simulink model "Signal_Generator"  (R2017a)
settings: Solver=VariableStepAuto  StartTime=0.0  StopTime=0.001  RelTol=1e-3
libraries: dspbuff3 x2
settings Model: Creator=Alam  LastModifiedBy=aparih

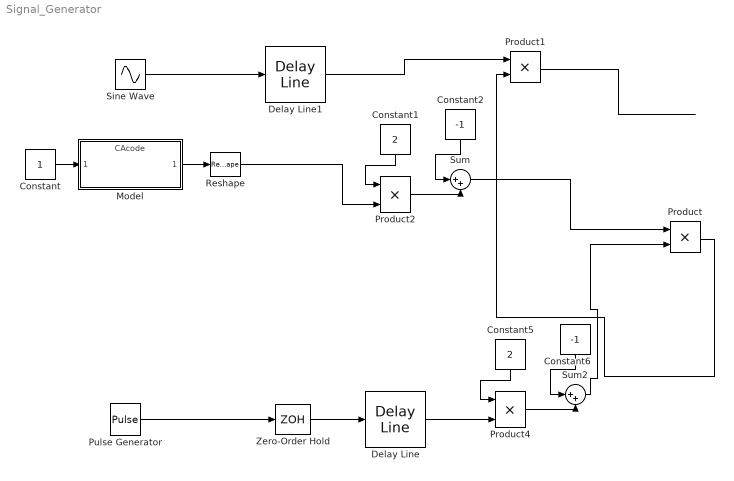
== system Signal_Generator ==
  Constant : Constant
  Constant1 : Constant  Value=2
  Constant2 : Constant  Value=-1
  Constant5 : Constant  Value=2
  Constant6 : Constant  Value=-1
  Delay Line : dspbuff3/Delay Line  siz=65536  ic=0  directfeed=off  enable_output=off  hold_output=off  OutputFrames=off
      settings: SourceProductName=DSP System Toolbox  SourceProductBaseCode=DS
  Delay Line1 : dspbuff3/Delay Line  siz=65536  ic=0  directfeed=off  enable_output=off  hold_output=off  OutputFrames=off
      settings: SourceProductName=DSP System Toolbox  SourceProductBaseCode=DS
  Model : ModelReference  ModelNameDialog=CAcode.mdl  SimulationMode=Normal  ModelReferenceVersion=1.40
  Product{,1..2,4} (4 alike) : Product
  Pulse Generator : DiscretePulseGenerator  PulseType=Time based  Period=0.0001  PulseWidth=50
  Reshape : Reshape  OutputDimensionality=Column vector (2-D)
  Sine Wave : Sin  Frequency=2*pi*9548000  Phase=pi/2  SampleTime=1.52587891e-8
  Sum : Sum  Inputs=|++
  Sum2 : Sum  Inputs=|++
  Zero-Order Hold : ZeroOrderHold  SampleTime=1.52587891e-8
  wires:
  Constant/1 -> Model/1
  Model/1 -> Reshape/1
  Constant1/1 -> Product2/1
  Product2/1 -> Sum/2
  Constant2/1 -> Sum/1
  Reshape/1 -> Product2/2
  Sine Wave/1 -> Delay Line1/1
  Sum2/1 -> Product/2
  Sum/1 -> Product/1
  Product/1 -> Product1/2
  Product1/1 -> ?
  Pulse Generator/1 -> Zero-Order Hold/1
  Constant6/1 -> Sum2/1
  Product4/1 -> Sum2/2
  Constant5/1 -> Product4/1
  Zero-Order Hold/1 -> Delay Line/1
  Delay Line/1 -> Product4/2
  Delay Line1/1 -> Product1/1
